simulink model "zero_cross_angle"  (R2022b)
settings: Solver=VariableStepAuto  StartTime=0.0  StopTime=0.08  MaxStep=1e-6  RelTol=1e-3
libraries: spsThyristorLib x4, spsVoltageMeasurementLib x3, spsACVoltageSourceLib x1, spsSeriesRLCBranchLib x1, dspswit3 x1, spsUniversalBridgeLib x1, sps_lib x1
settings Model: Creator=Dell  LastModifiedBy=Dell

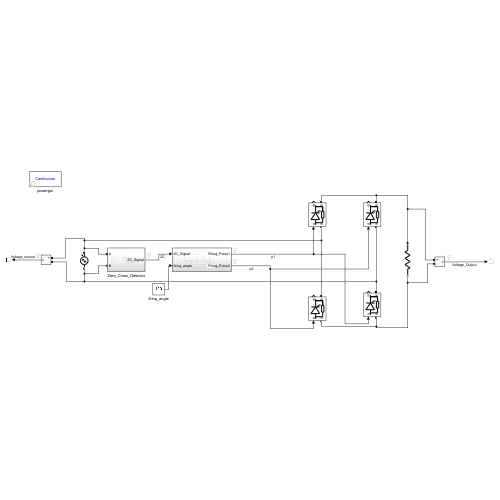
[thumbnail: Simulink's stored preview of the top-level diagram]
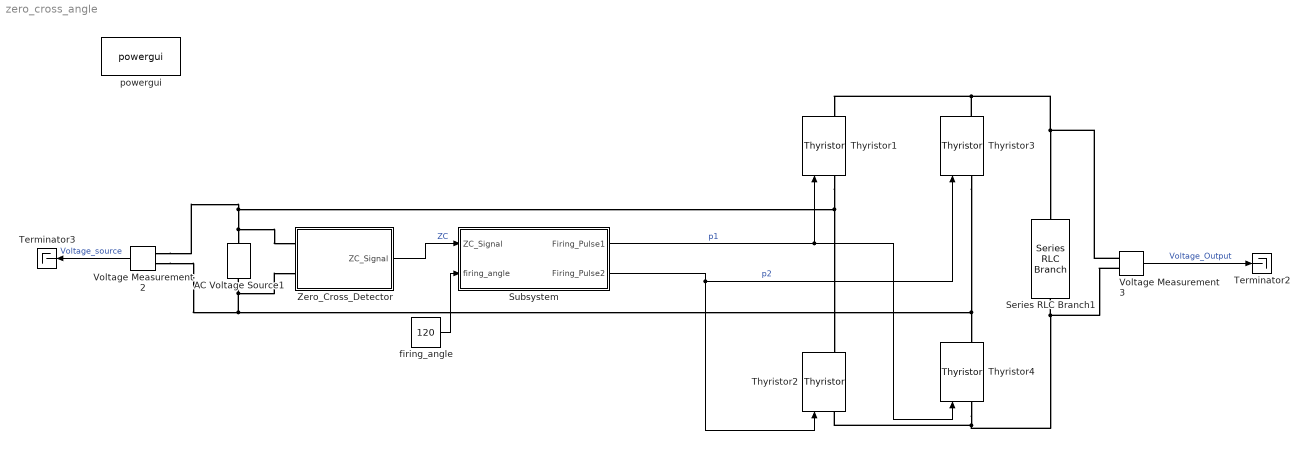
== system zero_cross_angle ==
  AC Voltage Source1 : spsACVoltageSourceLib/AC Voltage Source  Amplitude=220*sqrt(2)  Phase=0  Frequency=50  SampleTime=0  Measurements=None  BusType=swing  Pref=10e3  Qref=0  Qmin=-inf  Qmax=+inf
  Series RLC Branch1 : spsSeriesRLCBranchLib/Series RLC Branch  LConnTagsString=__new0  RConnTagsString=__new0  BranchType=R  Resistance=50  Inductance=1e-3  SetiL0=off  InitialCurrent=0  Capacitance=1e-6  Setx0=off  InitialVoltage=0  Measurements=None
  Subsystem : Subsystem
  Terminator2 : Terminator
  Terminator3 : Terminator
  Thyristor{1..4} (4 alike) : spsThyristorLib/Thyristor  Ron=0.001  Lon=0  Vf=0.8  IC=0  Rs=500  Cs=250e-9  Measurements=on
  Voltage Measurement2 : spsVoltageMeasurementLib/Voltage Measurement  PhasorSimulation=off  OutputType=Complex  PSBequivalent=0
  Voltage Measurement3 : spsVoltageMeasurementLib/Voltage Measurement  PhasorSimulation=off  OutputType=Complex  PSBequivalent=0
  Zero_Cross_Detector : Subsystem
  firing_angle : Constant  Value=120
  powergui : sps_lib/powergui  Priority=1  SimulationMode=Continuous  SampleTime=50e-6  frequency=60  Iterations=50  frequencyindice=50  Pbase=100e6  ErrMax=1e-4  UnitsV=kV  UnitsW=MW  buscounter=0  FunctionMessages=off  echomessages=off  EnableUseOfTLC=off  CurrentSourceSwitches=off  DisableSnubberDevices=off  DisableRonSwitches=off  DisableVfSwitches=off  DisplayEquations=off  AutomaticDiscreteSolvers=off  SolverType=Tustin/Backward Euler (TBE)  Interpol=off  ExternalGateDelay=off  methode=off  Ts=100  x0status=blocks  SPID=on  SwTol=0  HookPort=off  NonlinearTolerance=1e-4  nMaxIteration=100  ContinueOnMaxIteration=off  RestoreLinks=warning  ResistiveCurrentMeasurement=off  Frange=[0:2:500]  Ylog=off  Xlog=on  ShowGrid=off  save=off  variable=ZData  structure=0  ZoomFFT=off  StartTime=0.0  cycles=1  DisplayStyle=1  fundamental=60  FreqAxis=off  MaxFrequency=1000  frequencyindicesteady=1  RmsSteady=1  display=off
  wires:
  Voltage Measurement3/1 -> Terminator2/1  "Voltage_Output"
  Voltage Measurement2/1 -> Terminator3/1  "Voltage_source"
  Zero_Cross_Detector/1(ZC_Signal) -> Subsystem/1(ZC_Signal)  "ZC"
  Subsystem/1(Firing_Pulse1) -> Thyristor4/1, Thyristor1/1  "p1"
  Subsystem/2(Firing_Pulse2) -> Thyristor3/1, Thyristor2/1  "p2"
  firing_angle/1 -> Subsystem/2(firing_angle)
  connections:
  Voltage Measurement2/LConn1 -- Zero_Cross_Detector/LConn1 -- AC Voltage Source1/RConn1 -- Thyristor1/LConn1 -- Thyristor2/RConn1
  Voltage Measurement2/LConn2 -- Thyristor3/LConn1 -- Thyristor4/RConn1 -- Zero_Cross_Detector/LConn2 -- AC Voltage Source1/LConn1
  Voltage Measurement3/LConn1 -- Series RLC Branch1/LConn1 -- Thyristor3/RConn1 -- Thyristor1/RConn1
  Voltage Measurement3/LConn2 -- Thyristor2/LConn1 -- Thyristor4/LConn1 -- Series RLC Branch1/RConn1

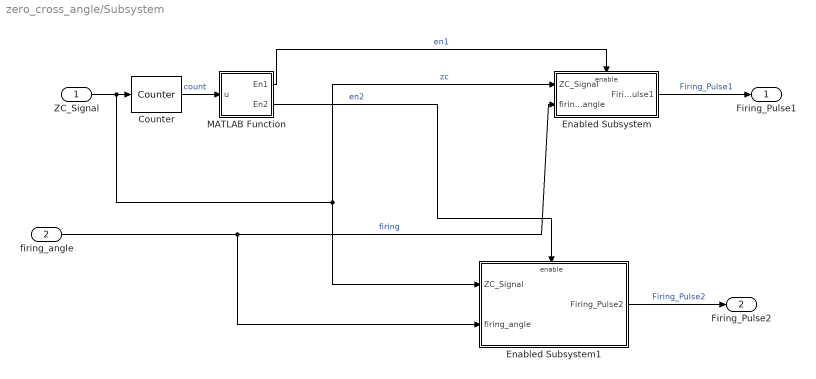
== system zero_cross_angle/Subsystem ==
  ZC_Signal : Inport
  firing_angle : Inport  Port=2
  Counter : dspswit3/Counter  Direction=Up  CountEvent=Rising edge  CounterSize=User defined  MaxCount=255  InitialCount=0  Output=Count  HitValue=32  ResetInput=off  SamplesPerFrame=1  Ts=1  CntDtype=double  HitDtype=Logical
  Enabled Subsystem : Subsystem  TreatAsAtomicUnit=on
  Enabled Subsystem1 : Subsystem  TreatAsAtomicUnit=on
  MATLAB Function : MATLAB Function  TreatAsAtomicUnit=on
  Firing_Pulse1 : Outport
  Firing_Pulse2 : Outport  Port=2
  wires:
  ZC_Signal/1 -> Enabled Subsystem1/1(ZC_Signal), Enabled Subsystem/1(ZC_Signal), Counter/1  "zc"
  Counter/1 -> MATLAB Function/1(u)  "count"
  Enabled Subsystem1/1(Firing_Pulse2) -> Firing_Pulse2/1  "Firing_Pulse2"
  Enabled Subsystem/1(Firing_Pulse1) -> Firing_Pulse1/1  "Firing_Pulse1"
  MATLAB Function/1(En1) -> Enabled Subsystem/Enable  "en1"
  MATLAB Function/2(En2) -> Enabled Subsystem1/Enable  "en2"
  firing_angle/1 -> Enabled Subsystem1/2(firing_angle), Enabled Subsystem/2(firing_angle)  "firing"

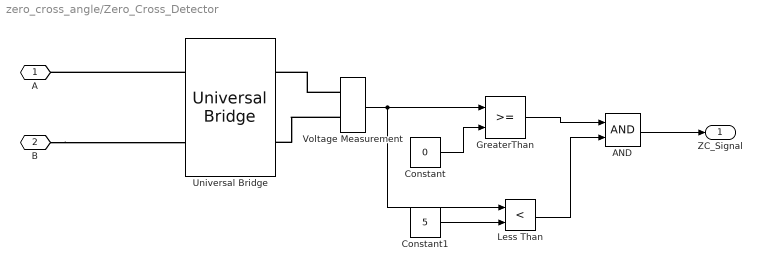
== system zero_cross_angle/Zero_Cross_Detector ==
  AND : Logic  AllPortsSameDT=off  OutDataTypeStr=boolean
  Constant : Constant  Value=0
  Constant1 : Constant  Value=5
  GreaterThan : RelationalOperator  OutDataTypeStr=boolean  RndMeth=Simplest  InputSameDT=off
  Less Than : RelationalOperator  Operator=<  OutDataTypeStr=boolean  RndMeth=Simplest  InputSameDT=off
  Universal Bridge : spsUniversalBridgeLib/Universal Bridge  Arms=2  SnubberResistance=1e5  SnubberCapacitance=inf  Device=Diodes  Ron=1e-3  Lon=0  ForwardVoltages="[  0  0  ]"  ForwardVoltage=0  GTOparameters=[ 10e-6 , 20e-6 ]  IGBTparameters=[ 1e-6 , 2e-6 ]  Measurements=None  Measurements_2=None  converterType=Rectifier
  Voltage Measurement : spsVoltageMeasurementLib/Voltage Measurement  PhasorSimulation=off  OutputType=Complex  PSBequivalent=0
  A : PMIOPort  Side=Left
  B : PMIOPort  Port=2  Side=Left
  ZC_Signal : Outport
  wires:
  Voltage Measurement/1 -> GreaterThan/1, Less Than/1
  Constant/1 -> GreaterThan/2
  Constant1/1 -> Less Than/2
  GreaterThan/1 -> AND/1
  Less Than/1 -> AND/2
  AND/1 -> ZC_Signal/1
  connections:
  Universal Bridge/LConn1 -- A/RConn1
  B/RConn1 -- Universal Bridge/LConn2
  Voltage Measurement/LConn1 -- Universal Bridge/RConn1
  Voltage Measurement/LConn2 -- Universal Bridge/RConn2

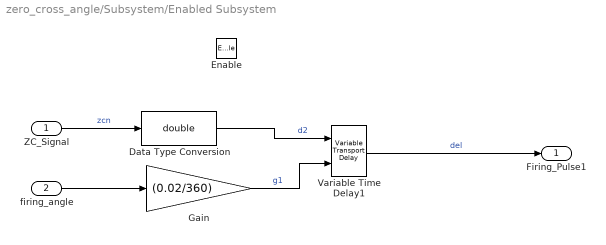
== system zero_cross_angle/Subsystem/Enabled Subsystem ==
  ZC_Signal : Inport
  firing_angle : Inport  Port=2
  Enable : EnablePort
  Data Type Conversion : DataTypeConversion  OutDataTypeStr=double  SaturateOnIntegerOverflow=off  RndMeth=Floor
  Gain : Gain  Gain=(0.02/360)
  Variable Time Delay1 : VariableTransportDelay  MaximumDelay=10  ZeroDelay=on
  Firing_Pulse1 : Outport
  wires:
  ZC_Signal/1 -> Data Type Conversion/1  "zcn"
  firing_angle/1 -> Gain/1
  Variable Time Delay1/1 -> Firing_Pulse1/1  "del"
  Data Type Conversion/1 -> Variable Time Delay1/1  "d2"
  Gain/1 -> Variable Time Delay1/2  "g1"

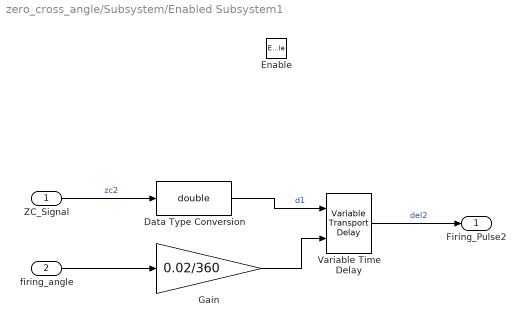
== system zero_cross_angle/Subsystem/Enabled Subsystem1 ==
  ZC_Signal : Inport
  firing_angle : Inport  Port=2
  Enable : EnablePort
  Data Type Conversion : DataTypeConversion  OutDataTypeStr=double  SaturateOnIntegerOverflow=off  RndMeth=Floor
  Gain : Gain  Gain=0.02/360
  Variable Time Delay : VariableTransportDelay  MaximumDelay=10  ZeroDelay=on
  Firing_Pulse2 : Outport
  wires:
  ZC_Signal/1 -> Data Type Conversion/1  "zc2"
  Data Type Conversion/1 -> Variable Time Delay/1  "d1"
  firing_angle/1 -> Gain/1
  Gain/1 -> Variable Time Delay/2
  Variable Time Delay/1 -> Firing_Pulse2/1  "del2"

== matlab function zero_cross_angle/Subsystem/MATLAB Function ==
  data: u input; En1 output; En2 output
function[En1, En2] = fcn(u)
En1=0;
En2=0;
if mod(u,2) == 0
    En1=1;
    En2=0;
elseif mod(u,2) == 1
    En1=0;
    En2=1;
end
